simulink model "AKZ_Gen"  (Simulink 4.00)
settings: Solver=ode23tb  StartTime=0.0  StopTime=0.5  MaxStep=1e-4  RelTol=1e-3
InitFcn:
  | powericon('psbinitsys',bdroot);
libraries: powerlib2 x8, powerlib_extras x4, simulink_extras x1
settings Model: BlockReductionOpt=off

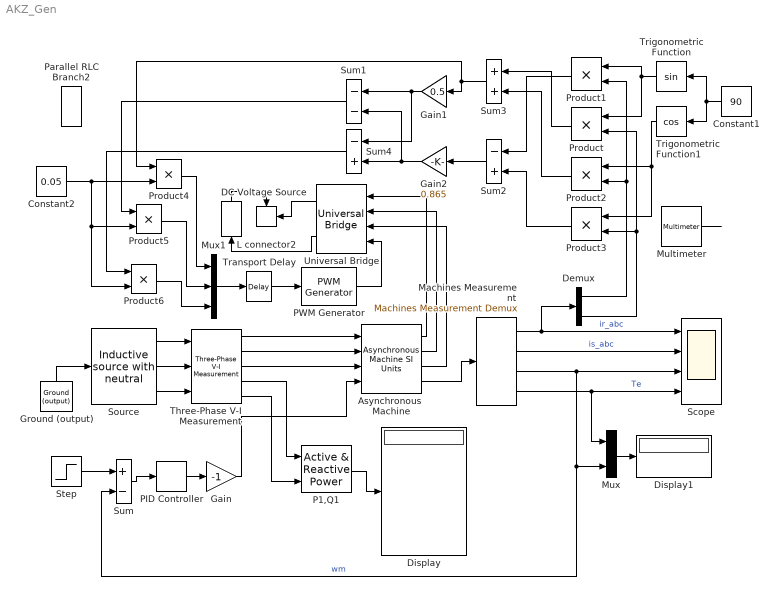
== system AKZ_Gen ==
  "Asynchronous  Machine " : powerlib2/Machines/Asynchronous Machine SI Units  Tag=PoWeRsYsTeMbLoCk  rotType=Wound  ctrl=Stationary  x1=[2e5, 380 50 ]  x2="[ 0.435  2.0e-3 ]"  x3="[ 0.00816  2.0e-3 ]"  x4=69.31e-3  x5="[ 0.089  0  2 ]"  x6="[ 1,0   0,0,0   0,0,0 ]"  PSBOutputType=1110  iounits=1
  Constant1 : Constant  Orientation=left  Value=90
  Constant2 : Constant  Value=0.05
  DC Voltage Source : powerlib2/Electrical Sources/DC Voltage Source  Tag=PoWeRsYsTeMbLoCk  Description=source block  Orientation=up  V=20  mesure=None  PSBOutputType=1
  Demux : Demux  Outputs=2  BusSelectionMode=off
  Display : Display
      settings: Format=short
  Display1 : Display
      settings: Format=short
  Gain : Gain  Gain=-1  Multiplication=Element-wise(K.*u)  SaturateOnIntegerOverflow=on
  Gain1 : Gain  Orientation=left  Gain=0.5  Multiplication=Element-wise(K.*u)  SaturateOnIntegerOverflow=on
  Gain2 : Gain  Orientation=left  Gain=0.865  Multiplication=Element-wise(K.*u)  SaturateOnIntegerOverflow=on
  Ground (output) : powerlib2/Connectors/Ground (output)  Tag=PoWeRsYsTeMbLoCk  Orientation=up  PSBOutputType=1
  L connector2 : powerlib2/Connectors/L connector  Tag=PoWeRsYsTeMbLoCk  Orientation=left
  Machines Measurement : powerlib2/Machines/Machines Measurement Demux  machType=Asynchronous  ssm1=on  ssm2=on  ssm3=on  ssm4=on  ssm5=on  ssm6=on  sm1=on  sm2=on  sm3=on  sm4=on  sm5=on  sm6=on  sm7=on  sm8=on  sm9=on  sm10=on  sm11=on  asm1=off  asm2=on  asm3=off  asm4=off  asm5=on  asm6=off  asm7=off  asm8=off  asm9=on  asm10=on  asm11=off  pmsm1=on  pmsm2=on  pmsm3=on  pmsm4=on  pmsm5=on  pmsm6=on  lastType=1
  Multimeter : powerlib2/Measurements/Multimeter  Tag=PoWeRsYsTeMmEaSuReMeNt  sel=[1 10]  L=15  Gain=[1 1]  yselected=[201,4.1000244140625000e+001;101,4.1000244140625000e+001]  PSBOutputType=1  PSBequivalent=0  AxesSetting=[0,0.1,-100,100]  Display=0  SavedBlockNames=-11
  Mux : Mux  Inputs=2
      settings: DisplayOption=none
  Mux1 : Mux  Inputs=3
  P1,Q1 : powerlib_extras/Measurements/Active & Reactive Power  f1=50
  PID Controller : simulink_extras/Additional Linear/PID Controller  P=10  I=100  D=0
  PWM Generator : powerlib_extras/Control  Blocks/PWM Generator  GeneratorMode="3-arm  bridge (6 pulses)"  Fc=100  Internal=off  mIndex=0.4  Freq=60  Phase=0
  Parallel RLC Branch2 : powerlib2/Elements/Parallel RLC Branch  Tag=PoWeRsYsTeMbLoCk  Orientation=up  a=10e5  b=1e-1  c=0  mesure=None  PSBOutputType=1
  Product{,1..3} (4 alike) : Product  Orientation=left  Inputs=2  Multiplication=Element-wise(.*)  SaturateOnIntegerOverflow=on
  Product4 : Product  Inputs=2  Multiplication=Element-wise(.*)  SaturateOnIntegerOverflow=on
  Product5 : Product  Inputs=2  Multiplication=Element-wise(.*)  SaturateOnIntegerOverflow=on
  Product6 : Product  Inputs=2  Multiplication=Element-wise(.*)  SaturateOnIntegerOverflow=on
  Scope : Scope  NumInputPorts=4
      settings: TimeRange=auto  YMin=-400~-400~0~-600  YMax=300~400~200~100  SaveToWorkspace=off  SaveName=ScopeData  MaxDataPoints=5000
  Source : powerlib_extras/Three-Phase Library/Inductive source with neutral  V=310  Phi=0  F=50  R=0.024  L=0
  Step : Step  Time=0  Before=0  After=160  SampleTime=0
  Sum : Sum  Inputs=+-  SaturateOnIntegerOverflow=on
  Sum1 : Sum  Orientation=left  Inputs=--  SaturateOnIntegerOverflow=on
  Sum2 : Sum  Orientation=left  Inputs=-+  SaturateOnIntegerOverflow=on
  Sum3 : Sum  Orientation=left  Inputs=++  SaturateOnIntegerOverflow=on
  Sum4 : Sum  Orientation=left  Inputs=-+  SaturateOnIntegerOverflow=on
  Three-Phase V-I Measurement : powerlib_extras/Measurements/Three-Phase V-I Measurement  Vpu=off  Vbase=500e3  Ppu=off  Pbase=100e6
  Transport Delay : TransportDelay  DelayTime=1e-4  InitialInput=0  BufferSize=1024  PadeOrder=0
  Trigonometric Function : Trigonometry  Orientation=left  Operator=sin  OutputSignalType=real
  Trigonometric Function1 : Trigonometry  Orientation=left  Operator=cos  OutputSignalType=real
  Universal Bridge : powerlib2/Power Electronics/Universal Bridge  Tag=PoWeRsYsTeMbLoCk  Orientation=left  arms=3  confi=ABC as input terminals  injcc=1e5  cf=inf  device=MOSFET / Diodes  Ron=1e-1  Lon=0  VFs="[  0.8  0.8  ]"  Vf=0  gtoparameters=[ 10e-6 , 20e-6 ]  igbtparameters=[ 1e-6 , 2e-6 ]  mesure=All voltages and currents  PSBOutputType=111
  wires:
  "Asynchronous  Machine "/4 -> Machines Measurement/1
  Source/1 -> Three-Phase V-I Measurement/1
  Source/2 -> Three-Phase V-I Measurement/2
  Source/3 -> Three-Phase V-I Measurement/3
  Three-Phase V-I Measurement/1 -> "Asynchronous  Machine "/1
  Three-Phase V-I Measurement/2 -> "Asynchronous  Machine "/2
  Three-Phase V-I Measurement/3 -> "Asynchronous  Machine "/3
  Three-Phase V-I Measurement/4 -> P1,Q1/1
  Three-Phase V-I Measurement/5 -> P1,Q1/2
  P1,Q1/1 -> Display/1
  Machines Measurement/1 -> Scope/1, Demux/1  "ir_abc"
  Ground (output)/1 -> Source/1
  Machines Measurement/2 -> Scope/2  "is_abc"
  Machines Measurement/3 -> Mux/2, Sum/2, Scope/3  "wm"
  Machines Measurement/4 -> Scope/4, Mux/1  "Te"
  Mux/1 -> Display1/1
  Step/1 -> Sum/1
  Sum/1 -> PID Controller/1
  PID Controller/1 -> Gain/1
  Gain/1 -> "Asynchronous  Machine "/4
  Constant1/1 -> Trigonometric Function/1, Trigonometric Function1/1
  Trigonometric Function/1 -> Product1/1, Product/1
  Trigonometric Function1/1 -> Product2/1, Product3/1
  Demux/1 -> Product1/2, Product2/2
  Demux/2 -> Product/2, Product3/2
  Product1/1 -> Sum2/1
  Product3/1 -> Sum2/2
  Product/1 -> Sum3/1
  Product2/1 -> Sum3/2
  Gain1/1 -> Sum1/1, Sum4/1
  Gain2/1 -> Sum1/2, Sum4/2
  Sum3/1 -> Gain1/1, Product4/1
  Sum2/1 -> Gain2/1
  Sum1/1 -> Product5/1
  Sum4/1 -> Product6/1
  Universal Bridge/2 -> DC Voltage Source/1
  Universal Bridge/1 -> L connector2/1
  DC Voltage Source/1 -> L connector2/Enable
  Product4/1 -> Mux1/1
  Product5/1 -> Mux1/2
  Product6/1 -> Mux1/3
  PWM Generator/1 -> Universal Bridge/4
  Multimeter/1 -> ?
  Mux1/1 -> Transport Delay/1
  Transport Delay/1 -> PWM Generator/1
  Constant2/1 -> Product4/2, Product5/2, Product6/2
  "Asynchronous  Machine "/1 -> Universal Bridge/1
  "Asynchronous  Machine "/2 -> Universal Bridge/2
  "Asynchronous  Machine "/3 -> Universal Bridge/3
